simulink model "cont"  (R2021b)
settings: Solver=VariableStepAuto  StartTime=0.0  StopTime=10.0  RelTol=1e-3
values from neighbouring files (symbols this model uses):
  A = sysest.A    [main.m]
  B = sysest.B    [main.m]
undefined symbols (not defined in the file or in its folder): k2, Kr2, sigbuilder_block, sysest
libraries: simulink_extras x2
settings Model: Creator=jesuc  LastModifiedBy=alpre

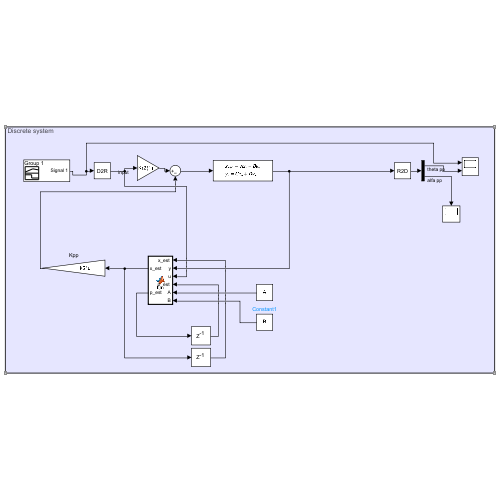
[thumbnail: Simulink's stored preview of the top-level diagram]
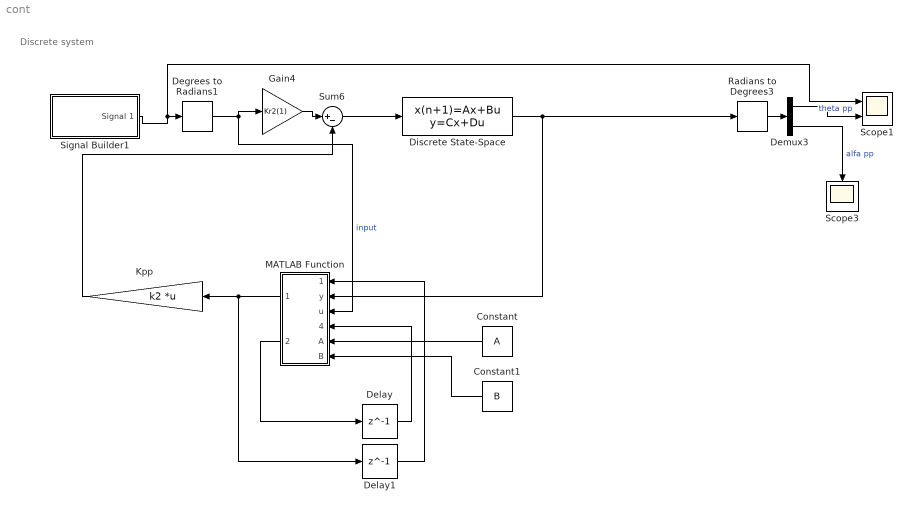
== system cont ==
  note: Discrete system
  Constant : Constant  Value=A
  Constant1 : Constant  Value=B
  Degrees to Radians1 : simulink_extras/Transformations/Degrees to Radians
  Delay : Delay  DelayLength=1  InitialCondition=eye(4)
  Delay1 : Delay  DelayLength=1  InitialCondition=0
  Demux3 : Demux  Outputs=2
  Discrete State-Space : DiscreteStateSpace  A=sysest.A  B=sysest.B  C=sysest.C  D=sysest.D  SampleTime=0.002
  Gain4 : Gain  Gain=Kr2(1)
  Kpp : Gain  Gain=k2  Multiplication=Matrix(K*u)
  MATLAB Function : MATLAB Function  TreatAsAtomicUnit=on
  Radians to Degrees3 : simulink_extras/Transformations/Radians to Degrees
  Scope1 : Scope  NumInputPorts=2
  Scope3 : Scope
  Signal Builder1 : Subsystem  Tag=STV Subsys  LoadFcn=sigbuilder_block('load');  StartFcn=sigbuilder_block('start');  StopFcn=sigbuilder_block('stop');  ClipboardFcn=sigbuilder_block('clipboard');  mask(Sigbuilder block){tuvar=[0:10]}
      mask help: Simulink:masks:SigbuilderBlock_MD
      mask init:
      | if ~strcmp(get_param(bdroot(gcbh),'SimulationStatus'),'stopped') tuvar = sigbuilder_block('maskInit'); end
      settings: CopyFcn=sigbuilder_block('copy');  DeleteFcn=sigbuilder_block('delete');  ModelCloseFcn=sigbuilder_block('modelClose');  PreSaveFcn=sigbuilder_block('preSave');  PauseFcn=sigbuilder_block('pause');  ContinueFcn=sigbuilder_block('continue');  NameChangeFcn=sigbuilder_block('namechange');  OpenFcn=sigbuilder_block('open',[437.6 199.2 550.4 400 ]);  CloseFcn=sigbuilder_block('close');
      mask Display: plot(0, 0, 100, 100,[2, 2, 32, 32, 2], [68, 8, 8, 68, 68],[32, 2], [38, 38], [32, 19, 2],[53, 60, 44], [32, 17, 17, 2],[16, 16, 31, 31]);txt = getActiveGroup(gcbh);text(2, 100, txt,'verticalAlignment', 'top');
  Sum6 : Sum  Inputs=|+-
  wires:
  Demux3/1 -> Scope1/2  "theta pp"
  Sum6/1 -> Discrete State-Space/1
  Signal Builder1/1(Signal 1) -> Scope1/1, Degrees to Radians1/1
  Discrete State-Space/1 -> MATLAB Function/2(y), Radians to Degrees3/1
  Radians to Degrees3/1 -> Demux3/1
  Demux3/2 -> Scope3/1  "alfa pp"
  Degrees to Radians1/1 -> MATLAB Function/3(u), Gain4/1  "input"
  Kpp/1 -> Sum6/2
  Gain4/1 -> Sum6/1
  MATLAB Function/2(p_est) -> Delay/1
  Delay/1 -> MATLAB Function/4("p_est ")
  MATLAB Function/1(x_est) -> Kpp/1, Delay1/1
  Constant/1 -> MATLAB Function/5(A)
  Constant1/1 -> MATLAB Function/6(B)
  Delay1/1 -> MATLAB Function/1("x_est ")

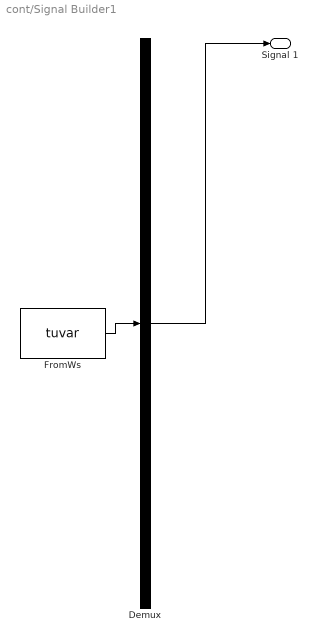
== system cont/Signal Builder1 ==
  Demux : Demux  Tag=STV Demux  Outputs=1
      settings: DisplayOption=none
  FromWs : FromWorkspace  Tag=STV FromWs  VariableName=tuvar
      SigBuilderData=|
      | common.afterFinalStr = 'Extrapolate'
      | common.sampleTime = 0
      | dataSet.timeRange = [0 10]
      | dataSet.name = 'Group 1'
      | sbobj.Groups.Name = 'Group 1'
      | sbobj.Groups.Signals.Name = 'Signal 1'
      | sbobj.Groups.Signals.XData = [0 1 1 3 3 5 5 7 7 8.5 8.5 10]
      | sbobj.Groups.Signals.YData = [0.005 0.005 40 40 15 15 -30 -30 0 0 23 23]
  Signal 1 : Outport  Tag=STV Outport
  wires:
  Demux/1 -> Signal 1/1
  FromWs/1 -> Demux/1

== matlab function cont/MATLAB Function ==
  data: x_est input; y input; u input; x_est output; p_est input; p_est output; A input; B input
function [x_est,p_est] = fcn(x_est,y,u,p_est, A,B)
% Initialize state transition matrix
% Measurement matrix
H = [ 1 0 0 0; 0  0 1 0 ];
Q = eye(4);
R = 10* eye(4);

% Predicted state and covariance
x_prd = A * x_est + B* u;
p_prd = A * p_est * A' + Q;
% Estimation
S = p_prd'  + R;
B = p_prd';
klm_gain = (S \ B)';
% Estimated state and covariance
x_est = x_prd + klm_gain * (pinv(H)*y - x_prd);
p_est = p_prd - klm_gain  * p_prd;
% Compute the estimated measurements
end
